simulink model "readRegisterTest"  (R2015b)
settings: Solver=FixedStepDiscrete  StartTime=0.0  StopTime=inf  FixedStep=1/100  RelTol=1e-3
libraries: quadLibrary x1
settings Model: SimulationMode=external  ExtModeEnableFloating=off  ExtModeTrigDuration=100  Creator=Nik Descher  LastModifiedBy=Nik Descher
settings DataIOCC: LimitDataPoints=off
settings OptimizationCC: OptimizeModelRefInitCode=on  LifeSpan=1
settings HardwareCC: ProdBitPerPointer=32  ProdLargestAtomicInteger=Long  ProdLargestAtomicFloat=Double  ProdWordSize=32  ProdHWDeviceType=ARM Compatible->ARM Cortex
settings RTWCC: SystemTargetFile=realtime.tlc  GenerateMakefile=off  TemplateMakefile=realtime.tmf  Description=Run on Target Hardware  RTWVerbose=off
settings STFCustomTargetCC: TargetLibSuffix=.a  GenerateSampleERTMain=on  ConcurrentExecutionCompliant=off  GeneratePreprocessorConditionals=Use local settings  ERTCustomFileBanners=on  SupportNonInlinedSFcns=off  SupportVariableSizeSignals=on  MATLABClassNameForMDSCustomization=Simulink.SoftwareTarget.ERTCustomization  CPPClassGenCompliant=off  GRTInterface=off  SystemTargetFile=realtime.tlc
settings ERTTargetCC: GenerateSampleERTMain=on  ParMdlRefBuildCompliant=off  CompOptLevelCompliant=off  ConcurrentExecutionCompliant=off  CombineOutputUpdateFcns=off  ERTFirstTimeCompliant=off  SupportContinuousTime=on  SupportVariableSizeSignals=on  ModelStepFunctionPrototypeControlCompliant=off  CPPClassGenCompliant=off  UseToolchainInfoCompliant=off  ExtModeMexArgs='192.168.1.248' 0 17725  ERTSrcFileBannerTemplate=realtime_code_template.cgt  ERTHdrFileBannerTemplate=realtime_code_template.cgt  ERTDataSrcFileTemplate=realtime_code_template.cgt  ERTDataHdrFileTemplate=realtime_code_template.cgt  ERTCustomFileTemplate=realtime_file_process.tlc

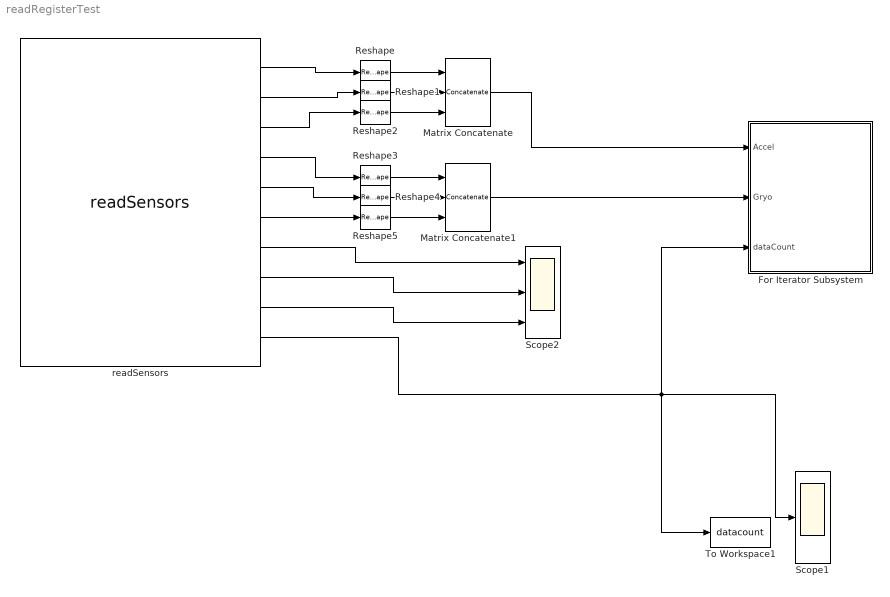
== system readRegisterTest ==
  For Iterator Subsystem : Subsystem  TreatAsAtomicUnit=on
  Matrix Concatenate : Concatenate  NumInputs=3  Mode=Multidimensional array
  Matrix Concatenate1 : Concatenate  NumInputs=3  Mode=Multidimensional array
  Reshape{,1..5} (6 alike) : Reshape  OutputDimensionality=Row vector (2-D)
  Scope1 : Scope
  Scope2 : Scope  NumInputPorts=3
  To Workspace1 : ToWorkspace  VariableName=datacount  SaveFormat=Structure With Time  SampleTime=-1
  readSensors : quadLibrary/readSensors
  wires:
  readSensors/1 -> Reshape/1
  readSensors/2 -> Reshape1/1
  readSensors/3 -> Reshape2/1
  readSensors/4 -> Reshape3/1
  readSensors/5 -> Reshape4/1
  readSensors/6 -> Reshape5/1
  Matrix Concatenate/1 -> For Iterator Subsystem/1(Accel)
  Matrix Concatenate1/1 -> For Iterator Subsystem/2(Gryo)
  Reshape/1 -> Matrix Concatenate/1
  Reshape1/1 -> Matrix Concatenate/2
  Reshape2/1 -> Matrix Concatenate/3
  Reshape3/1 -> Matrix Concatenate1/1
  Reshape4/1 -> Matrix Concatenate1/2
  Reshape5/1 -> Matrix Concatenate1/3
  readSensors/7 -> Scope2/1
  readSensors/8 -> Scope2/2
  readSensors/9 -> Scope2/3
  readSensors/10 -> For Iterator Subsystem/3(dataCount), To Workspace1/1, Scope1/1

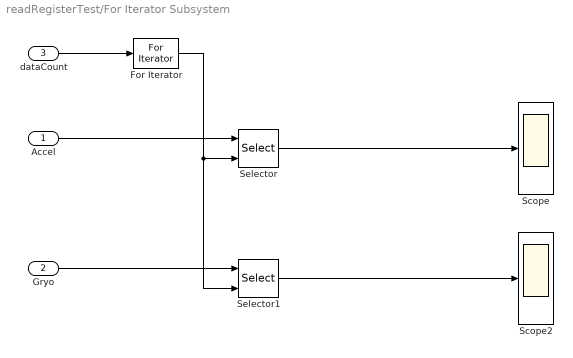
== system readRegisterTest/For Iterator Subsystem ==
  Accel : Inport
  Gryo : Inport  Port=2
  dataCount : Inport  Port=3
  For Iterator : ForIterator  IterationSource=external
  Scope : Scope
  Scope2 : Scope
  Selector : Selector  NumberOfDimensions=2  InputPortWidth=3  IndexOptions=Index vector (dialog),Index vector (port)  Indices=[1 2 3],1  OutputSizes=1,1
  Selector1 : Selector  NumberOfDimensions=2  InputPortWidth=3  IndexOptions=Index vector (dialog),Index vector (port)  Indices=[1 2 3],1  OutputSizes=1,1
  wires:
  dataCount/1 -> For Iterator/1
  Accel/1 -> Selector/1
  For Iterator/1 -> Selector1/2, Selector/2
  Selector/1 -> Scope/1
  Gryo/1 -> Selector1/1
  Selector1/1 -> Scope2/1
